simulink model "sem1_simul_motordc"  (R2022b)
settings: Solver=VariableStepAuto  StartTime=0.0  StopTime=10.0  RelTol=1e-3
values from neighbouring files (symbols this model uses):
  B = [0 ... (first row only)    [sem2_sol_EE.m]    (also in sem5_diseno_reg_pendulo_inv.m)
undefined symbols (not defined in the file or in its folder): J, Ke, Kt, La, Ra
settings Model: Creator=Celso  LastModifiedBy=Celso

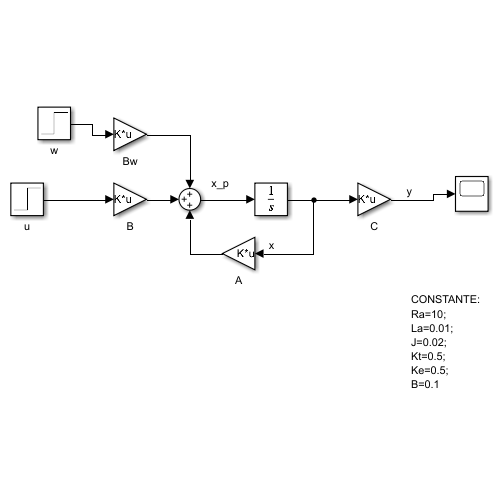
[thumbnail: Simulink's stored preview of the top-level diagram]
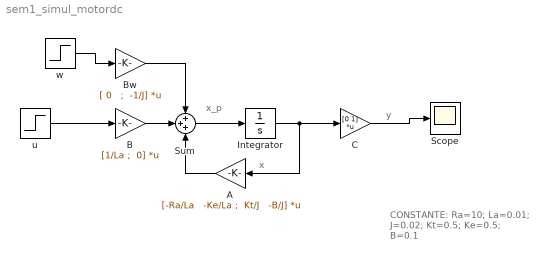
== system sem1_simul_motordc ==
  note: CONSTANTE:
      | Ra=10;
      | La=0.01;
      | J=0.02;
      | Kt=0.5;
      | Ke=0.5;
      | B=0.1
  note: y
  note: x_p
  note: x
  A : Gain  Gain="[-Ra/La   -Ke/La ;  Kt/J   -B/J]"  Multiplication=Matrix(K*u)
  B : Gain  Gain="[1/La ;  0]"  Multiplication=Matrix(K*u)
  Bw : Gain  Gain="[ 0   ;  -1/J]"  Multiplication=Matrix(K*u)
  C : Gain  Gain="[0   1]"  Multiplication=Matrix(K*u)
  Integrator : Integrator
  Scope : Scope
  Sum : Sum  Inputs=+++
  u : Step  Time=0  After=12  SampleTime=0
  w : Step  Time=5  SampleTime=0
  wires:
  u/1 -> B/1
  B/1 -> Sum/2
  A/1 -> Sum/3
  Bw/1 -> Sum/1
  Sum/1 -> Integrator/1
  Integrator/1 -> C/1, A/1
  w/1 -> Bw/1
  C/1 -> Scope/1
